simulink model "solution_simulinkModelMech"  (R2025b)
settings: Solver=VariableStepAuto  StartTime=0.0  StopTime=stopTime  MaxStep=1e-3  RelTol=1e-3
undefined symbols (not defined in the file): c, k, m, x0, x0_dot
settings Model: Creator=simom  LastModifiedBy=simom

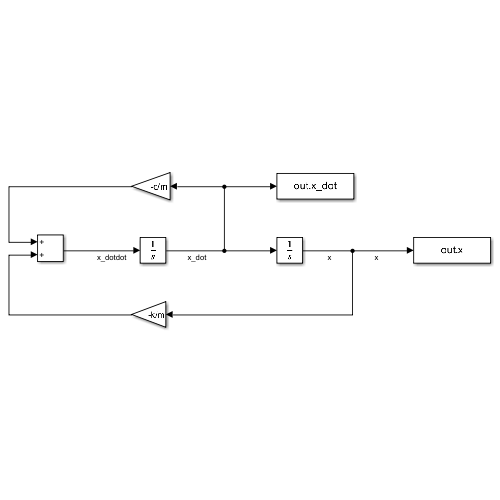
[thumbnail: Simulink's stored preview of the top-level diagram]
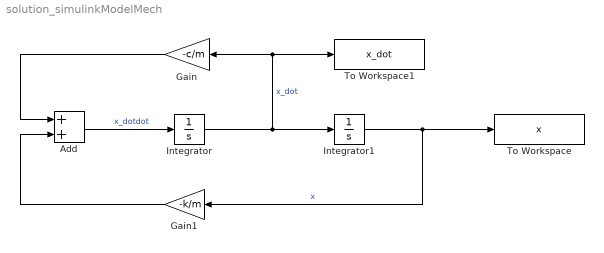
== system solution_simulinkModelMech ==
  Add : Sum
  Gain : Gain  Gain=-c/m
  Gain1 : Gain  Gain=-k/m
  Integrator : Integrator  InitialCondition=x0_dot
  Integrator1 : Integrator  InitialCondition=x0
  To Workspace : ToWorkspace  VariableName=x  SampleTime=-1
  To Workspace1 : ToWorkspace  VariableName=x_dot  SampleTime=-1
  wires:
  Add/1 -> Integrator/1  "x_dotdot"
  Integrator/1 -> To Workspace1/1, Gain/1, Integrator1/1  "x_dot"
  Integrator1/1 -> To Workspace/1, Gain1/1  "x"
  Gain/1 -> Add/1
  Gain1/1 -> Add/2
